simulink model "untitled1"  (R2022a)
settings: Solver=FixedStepAuto  StartTime=0.0  StopTime=1  RelTol=1e-3
libraries: simrfV2elements x1, simrfV2util1 x1, commdigbbndam3 x1, dspfdesign x1
settings Model: Creator=25671  LastModifiedBy=Administrator

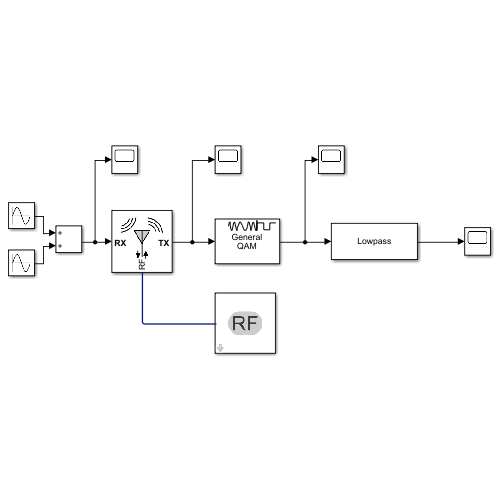
[thumbnail: Simulink's stored preview of the top-level diagram]
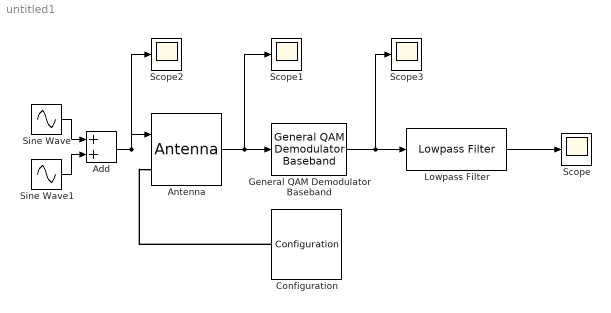
== system untitled1 ==
  Add : Sum
  Antenna : simrfV2elements/Antenna  AntennaSource=Isotropic radiator  PrevAppliedAntSource=Isotropic radiator  Gr=1 None  Zin=50  AntennaObj=antObj  InputIncWave=on  OutputRadWave=on  CarrierFreqInc=2.1 MHz  rArr=[180 0] deg  CarrierFreqRad=2.1 MHz  rDep=[0 0] deg  AddNoise=on  InternalGrounding=on  SparamRepresentationImp=Time domain (rationalfit)  FitTolImp=-40  AutoImpulseLengthImp=on  ImpulseLengthImp=1e-10 s
      settings: SourceProductBaseCode=RB
  Configuration : simrfV2util1/Configuration  AutoFreq=on  Tones=[2.1] GHz  Harmonics=[7]  NormalizeCarrierPower=on  SolverType=Auto  UseCCode=on  StepSize=1e-6 s  AddNoise=on  defaultRNG=on  Seed=0  Temperature=290.0 K  SolverDelFlag=0  AbsTol=1e-6  RelTol=1e-3  MaxIter=10  ErrorEstimationType=2-norm over all variables  EnableInterpFilter=on  HiddenFIRfilterControllerParam=on  SmallSignalApprox=off  AllSimFreqs=on  SimFreqs=[] Hz  SimFreqsInternal=[]  SamplesPerFrame=1
      settings: SourceProductBaseCode=RB
  General QAM Demodulator Baseband : commdigbbndam3/General QAM Demodulator Baseband  SigCon=[exp(2*pi*1i*[0:7]/8)]  OutType=Integer  DecType=Hard decision  VarSource=Dialog  Variance=1  outDtypeBit=Inherit via internal rule  outDtype=Inherit via internal rule  roundingMode=Floor  overflowMode=Wrap  OvFlMode=off  OvFlModeLastStrValue=off  sigConstWordLen=16  sigConstDataTypeStr=Inherit: Same word length as input  sigConstLastDataTypeStr=Inherit: Same word length as input  accum1WordLen=32  accum1FracLen=30  prodInWordLen=32  prodInFracLen=30  prodInDataTypeStr=Inherit: Same as accumulator 1  prodInLastDataTypeStr=Inherit: Same as accumulator 1  prodOutWordLen=32  prodOutFracLen=30  accum2WordLen=32  accum2FracLen=30  accum3WordLen=32  accum3FracLen=30  nsiWordLen=32  nsiFracLen=30  nsiDataTypeStr=Inherit: Same as accumulator 3  nsiLastDataTypeStr=Inherit: Same as accumulator 3  invn0WordLen=16  invn0FracLen=8  invn0DataTypeStr=Inherit: Same word length as input  invn0LastDataTypeStr=Inherit: Same word length as input  outputWordLen=32  outputFracLen=30
      settings: SourceProductBaseCode=CM
  Lowpass Filter : dspfdesign/Lowpass Filter  FilterType=FIR  DesignForMinimumOrder=on  FilterOrder=50  PassbandFrequency=8e3  StopbandFrequency=12e3  PassbandRipple=0.1  StopbandAttenuation=80  InheritSampleRate=off  SampleRate=44100  SimulateUsing=Interpreted execution  roundingMode=Floor  coeffsDataTypeStr=fixdt(1,16)
  Scope{,1..3} (4 alike) : Scope
  Sine Wave : Sin  Amplitude=0.5  Frequency=100  SampleTime=0
  Sine Wave1 : Sin  Amplitude=0.5  Frequency=10  SampleTime=0
  wires:
  General QAM Demodulator Baseband/1 -> Scope3/1, Lowpass Filter/1
  Lowpass Filter/1 -> Scope/1
  Antenna/1 -> Scope1/1, General QAM Demodulator Baseband/1
  Add/1 -> Scope2/1, Antenna/1
  Sine Wave/1 -> Add/1
  Sine Wave1/1 -> Add/2
  connections:
  Configuration/LConn1 -- Antenna/LConn1
